simulink model "ECE595_Part1_Project_Lidar_based_Motor_Control_Slave"  (R2017a)
settings: Solver=FixedStepDiscrete  StartTime=0.0  StopTime=10  FixedStep=dt  RelTol=1e-3
InitFcn:
  | mbd_s32k14_consistency_checks(bdroot(gcs));
model workspace (MAT data in the model file):
  MCOS : class17 (value not decoded)
undefined symbols (not defined in the file): A10, AD12, AD6, AD7, Aligned, B10, B8, B9, C10, C7, C8, C9, D1, D2, D8, Edge, External, G2, G3, G5, G6, H8, K10, K5, PTA1, PTA2, PTA3, PTB10, PTB11, PTB12, PTB8, PTB9, PTC10, PTC11, PTC14, PTC6, PTC7, PTD10, PTD11, PTD15, PTD16, PTD4, PTE4, PTE5, SpeedControllerIntegGain, SpeedControllerPropGain, TRGMUX_PDB_TRIG
libraries: mbd_s32k14_ec_toolbox x35, simulink x9
(part 2 of 2)

== system ECE595_Part1_Project_Lidar_based_Motor_Control_Slave/RX_Complete_Event/Switch Case Action Subsystem Data 4 ==
  Action Port : ActionPort  ActionType=case
  Constant : Constant  Value=800  OutDataTypeStr=int16
  Data Store Write : DataStoreWrite  DataStoreName=MotorSpeedReqFreemaster
  FCAN_Receive_ID_0x3FF : mbd_s32k14_ec_toolbox/S32K14x/Communication Blocks/Flex CAN Blocks/FCAN_Receive  can_instance=0  can_mode=Non-blocking  can_timeout_ms=0  can_mb_idx=14  can_extended_id=off  can_is_remote=off  can_id=3FF  can_msg_mask=FFFFFFFF  show_adv_opts=on  can_use_rxfifo=off  can_fd_enable=on
  wires:
  Constant/1 -> Data Store Write/1

== system ECE595_Part1_Project_Lidar_based_Motor_Control_Slave/RX_Complete_Event/Switch Case Action Subsystem Data 5 ==
  Action Port : ActionPort  ActionType=case
  Constant : Constant  Value=800  OutDataTypeStr=int16
  Data Store Write : DataStoreWrite  DataStoreName=MotorSpeedReqFreemaster
  FCAN_Receive_ID_0x3FF : mbd_s32k14_ec_toolbox/S32K14x/Communication Blocks/Flex CAN Blocks/FCAN_Receive  can_instance=0  can_mode=Non-blocking  can_timeout_ms=0  can_mb_idx=14  can_extended_id=off  can_is_remote=off  can_id=3FF  can_msg_mask=FFFFFFFF  show_adv_opts=on  can_use_rxfifo=off  can_fd_enable=on
  wires:
  Constant/1 -> Data Store Write/1

== system ECE595_Part1_Project_Lidar_based_Motor_Control_Slave/RX_Complete_Event/Switch Case Action Subsystem Data 6 ==
  Action Port : ActionPort  ActionType=case
  Constant : Constant  Value=800  OutDataTypeStr=int16
  Data Store Write : DataStoreWrite  DataStoreName=MotorSpeedReqFreemaster
  FCAN_Receive_ID_0x3FF : mbd_s32k14_ec_toolbox/S32K14x/Communication Blocks/Flex CAN Blocks/FCAN_Receive  can_instance=0  can_mode=Non-blocking  can_timeout_ms=0  can_mb_idx=14  can_extended_id=off  can_is_remote=off  can_id=3FF  can_msg_mask=FFFFFFFF  show_adv_opts=on  can_use_rxfifo=off  can_fd_enable=on
  wires:
  Constant/1 -> Data Store Write/1

== system ECE595_Part1_Project_Lidar_based_Motor_Control_Slave/RX_Complete_Event/Switch Case Action Subsystem Data 7 ==
  Action Port : ActionPort  ActionType=case
  Constant : Constant  Value=800  OutDataTypeStr=int16
  Data Store Write : DataStoreWrite  DataStoreName=MotorSpeedReqFreemaster
  FCAN_Receive_ID_0x3FF : mbd_s32k14_ec_toolbox/S32K14x/Communication Blocks/Flex CAN Blocks/FCAN_Receive  can_instance=0  can_mode=Non-blocking  can_timeout_ms=0  can_mb_idx=14  can_extended_id=off  can_is_remote=off  can_id=3FF  can_msg_mask=FFFFFFFF  show_adv_opts=on  can_use_rxfifo=off  can_fd_enable=on
  wires:
  Constant/1 -> Data Store Write/1

== system ECE595_Part1_Project_Lidar_based_Motor_Control_Slave/CalculateRPM/Actual Motor Speed Calculation/Calc_RPM1 ==
  note: Multiply by time constant to get Second
      | Mulitply by 60 to get Minute
      | Divide By State Changes to get Electrical RPM
      | Divide By Pole-Pair to get Mechanical RPM
  HallChangeSum : Inport
  Dir : Inport  Port=2
  GetDirection : Product  Inputs=**  OutDataTypeStr=int16  RndMeth=Zero
  State Changes to RPM Constant : Constant  Value=((1/(dt*250))*60)/(6*4)  OutDataTypeStr=uint16
  TransPerMin : Product  Inputs=**  OutDataTypeStr=uint16  RndMeth=Zero
  RPM : Outport
  wires:
  Dir/1 -> GetDirection/2
  GetDirection/1 -> RPM/1  "MotorSpeedRPM"
  State Changes to RPM Constant/1 -> TransPerMin/2
  HallChangeSum/1 -> TransPerMin/1
  TransPerMin/1 -> GetDirection/1

== system ECE595_Part1_Project_Lidar_based_Motor_Control_Slave/Event_Control/ControlEventLogic/HallChangeCount ==
  function : TriggerPort  TriggerType=function-call  VariantControl=Variant
  Constant5 : Constant  OutDataTypeStr=uint16
  Data Store Read : DataStoreRead  DataStoreName=HallStateChangeDelta
  Data Store Write : DataStoreWrite  DataStoreName=HallStateChangeDelta
  Function-Call Generator : simulink/Ports & Subsystems/Function-Call Generator  sample_time=-1  numberOfIterations=1
  Increment : Sum
  Call : Outport
  wires:
  Increment/1 -> Data Store Write/1
  Constant5/1 -> Increment/1
  Data Store Read/1 -> Increment/2
  Function-Call Generator/1 -> Call/1

== system ECE595_Part1_Project_Lidar_based_Motor_Control_Slave/Event_Control/ControlEventLogic/ToggleLED_HallA ==
  function : TriggerPort  TriggerType=function-call  VariantControl=Variant
  Data Store Read1 : DataStoreRead  DataStoreName=HallInputA
  Data Store Write1 : DataStoreWrite  DataStoreName=HallInputA
  Function-Call Generator : simulink/Ports & Subsystems/Function-Call Generator  sample_time=-1  numberOfIterations=1
  Logical Operator : Logic  Operator=NOT  AllPortsSameDT=off  OutDataTypeStr=boolean
  Call : Outport
  wires:
  Function-Call Generator/1 -> Call/1
  Data Store Read1/1 -> Logical Operator/1
  Logical Operator/1 -> Data Store Write1/1

== system ECE595_Part1_Project_Lidar_based_Motor_Control_Slave/Event_Control/ControlEventLogic/ToggleLED_HallB ==
  function : TriggerPort  TriggerType=function-call  VariantControl=Variant
  Data Store Read1 : DataStoreRead  DataStoreName=HallInputB
  Data Store Write1 : DataStoreWrite  DataStoreName=HallInputB
  Function-Call Generator : simulink/Ports & Subsystems/Function-Call Generator  sample_time=-1  numberOfIterations=1
  Logical Operator : Logic  Operator=NOT  AllPortsSameDT=off  OutDataTypeStr=boolean
  Call : Outport
  wires:
  Function-Call Generator/1 -> Call/1
  Data Store Read1/1 -> Logical Operator/1
  Logical Operator/1 -> Data Store Write1/1

== system ECE595_Part1_Project_Lidar_based_Motor_Control_Slave/Event_Control/ControlEventLogic/ToggleLED_HallC ==
  function : TriggerPort  TriggerType=function-call  VariantControl=Variant
  Data Store Read1 : DataStoreRead  DataStoreName=HallInputC
  Data Store Write1 : DataStoreWrite  DataStoreName=HallInputC
  Function-Call Generator : simulink/Ports & Subsystems/Function-Call Generator  sample_time=-1  numberOfIterations=1
  Logical Operator : Logic  Operator=NOT  AllPortsSameDT=off  OutDataTypeStr=boolean
  Call : Outport
  wires:
  Function-Call Generator/1 -> Call/1
  Data Store Read1/1 -> Logical Operator/1
  Logical Operator/1 -> Data Store Write1/1

== stateflow chart ECE595_Part1_Project_Lidar_based_Motor_Control_Slave/CalculateRPM/Actual Motor Speed Calculation/GatherNumberOfHallStateChanges ==
  (default) -> (junction 5)
  (junction 5) -> (junction 6) : {
      | 	HallChangesSum = HallChangesSum - StoreHallChanges[i];
      | 	StoreHallChanges[i] = HallChanges;
      | 	HallChangesSum = HallChangesSum + StoreHallChanges[i];
      | 	i++;
      | }
  (junction 6) -> (junction 22) [order 2] : {
      | 	HallChangeClear = 0;
      | }
  (junction 6) -> (junction 6) [order 1] : [i >= 250]
      | {i=0;}
  data: StoreHallChanges local uint8 size=[250]; HallChanges input; HallChangesSum output uint16; i local uint8; HallChangeClear output

== stateflow chart ECE595_Part1_Project_Lidar_based_Motor_Control_Slave/Control_Logic/FET pre-driver Initialization Sequence ==
  settings: sampleTime=0.500
  state A
  state B
  state C
  state C1
  state C2
  state D
  state E
  state F
    F -> F [order 1] : {index++;}
  state END
  (default) -> A : {enable=0;}
  A -> B : /*MASK0*/
      | {MPC_Data = 0x20;}
  B -> C : /*MASK1*/
      | {MPC_Data = 0x30;}
  C -> C1 : /*CLINT0*/
      | {MPC_Data = 0x6F;}
  C1 -> C2 : /*CLINT1*/
      | {MPC_Data = 0x7F;}
  C2 -> D : /*Mode*/
      | {MPC_Data  = 0x48;}
  D -> E : {MPC_Data = 0x00;
      | enable=1;}
  E -> F : {Charge_Bootstrap_Low_On;
      | index=0;}
  F -> END [order 1] : [index > 0]
      | {Charge_Bootstrap_All_Off;}
  END -> END : {Normal_Op;
      | MPC_Data = MPC_Cmd;}
  data: MPC_Data output uint16; enable output boolean; index local double; MPC_Cmd data_store_memory
  events: Charge_Bootstrap_Low_On output FUNCTION_CALL_EVENT; Charge_Bootstrap_All_Off output FUNCTION_CALL_EVENT; Normal_Op output FUNCTION_CALL_EVENT

== stateflow chart ECE595_Part1_Project_Lidar_based_Motor_Control_Slave/Event_Control/ControlPollingLogic ==
  state Logic1
    Logic1 -> (junction 25)
    (default) -> (junction 25)
    (junction 25) -> (junction 26) [order 1] : [(MotorSpeedRPM <= 100) && (MotorSpeedRPM >= -100)]
        | {Trigger;}
    (junction 25) -> (junction 28) [order 2]
    (junction 26) -> (junction 27)
    (junction 28) -> (junction 27)
  (default) -> Logic1
  data: MotorSpeedRPM input
  events: Trigger output FUNCTION_CALL_EVENT

== stateflow chart ECE595_Part1_Project_Lidar_based_Motor_Control_Slave/Event_Control/Init ==
  settings: sampleTime=0.500
  state A
  state B
  (default) -> A
  A -> B : {Init;
      | index=0;}
  B -> B
  data: index local double
  events: Init output FUNCTION_CALL_EVENT

== stateflow chart ECE595_Part1_Project_Lidar_based_Motor_Control_Slave/Trapezoidal_Commutation/CommutationTableLookup ==
  (junction 5) -> (junction 15) [order 1] : /*If Direction is Negative */
      | [Direction == -1]
  (default) -> (junction 5)
  (junction 15) -> (junction 14) : {
      |    Phase_A = ccwTable[HallState][0];
      |    Phase_B = ccwTable[HallState][1];
      |    Phase_C = ccwTable[HallState][2];
      | }
  (junction 5) -> (junction 6) [order 2] : {
      |    Phase_A = cwTable[HallState][0];
      |    Phase_B = cwTable[HallState][1];
      |    Phase_C = cwTable[HallState][2];
      | }
  (junction 6) -> (junction 14)
  data: cwTable constant uint8 size=[8 3] =[0 0 0; 2 1 0; 0 2 1; 2 0 1; 1 0 2; 0 1 2; 1 2 0; 0 0 0]; HallState input; Phase_A output uint8; Phase_B output uint8; Phase_C output uint8; ccwTable constant uint8 size=[8 3] =[0 0 0; 1 2 0; 0 1 2; 1 0 2; 2 0 1; 0 2 1; 2 1 0; 0 0 0]; Direction input

== stateflow chart ECE595_Part1_Project_Lidar_based_Motor_Control_Slave/Trapezoidal_Commutation/PhaseSwitchLogic ==
  settings: sampleTime=0.500
  note: Phase States:
      | 0 = NC
      | 1 = -Vdcb
      | 2 = +Vdcb
  (default) -> (junction 13)
  (junction 13) -> (junction 14) [order 1] : /*check for phase state 0 */
      | [Phase_A == 0]
      | /*set output for state 0 */
      | {Phase_A_HS = 0; Phase_A_LS =0;}
  (junction 13) -> (junction 17) [order 2]
  (junction 14) -> (junction 16)
  (junction 17) -> (junction 16) [order 1] : /*check for phase state 1 */
      | [Phase_A == 1]
      | /*set output for state 1 */
      | {Phase_A_HS = 0; Phase_A_LS = PWM_Duty_Cycle;}
  (junction 17) -> (junction 20) [order 2]
  (junction 16) -> (junction 19)
  (junction 20) -> (junction 19) [order 1] : /*check for phase state 2 */
      | [Phase_A == 2]
      | /*set output for state 2 */
      | {Phase_A_HS = 1000; Phase_A_LS = 0;}
  (junction 20) -> (junction 62) [order 2]
  (junction 19) -> (junction 23)
  (junction 62) -> (junction 23)
  (junction 23) -> (junction 22) [order 1] : /*check for phase state 0 */
      | [Phase_B == 0]
      | /*set output for state 0 */
      | {Phase_B_HS = 0; Phase_B_LS = 0;}
  (junction 23) -> (junction 26) [order 2]
  (junction 22) -> (junction 25)
  (junction 26) -> (junction 25) [order 1] : /*check for phase state 1 */
      | [Phase_B == 1]
      | /*set output for state 1 */
      | {Phase_B_HS = 0; Phase_B_LS = PWM_Duty_Cycle;}
  (junction 26) -> (junction 29) [order 2]
  (junction 25) -> (junction 28)
  (junction 29) -> (junction 28) [order 1] : /*check for phase state 2 */
      | [Phase_B == 2]
      | /*set output for state 2 */
      | {Phase_B_HS = 1000; Phase_B_LS = 0;}
  (junction 29) -> (junction 65) [order 2]
  (junction 28) -> (junction 49)
  (junction 65) -> (junction 49)
  (junction 49) -> (junction 48) [order 1] : /*check for phase state 0 */
      | [Phase_C == 0]
      | /*set output for state 0 */
      | {Phase_C_HS = 0; Phase_C_LS = 0;}
  (junction 49) -> (junction 51) [order 2]
  (junction 48) -> (junction 50)
  (junction 51) -> (junction 50) [order 1] : /*check for phase state 1 */
      | [Phase_C == 1]
      | /*set output for state 1 */
      | {Phase_C_HS = 0; Phase_C_LS = PWM_Duty_Cycle;}
  (junction 51) -> (junction 53) [order 2]
  (junction 50) -> (junction 52)
  (junction 53) -> (junction 52) [order 1] : /*check for phase state 2 */
      | [Phase_C == 2]
      | /*set output for state 2 */
      | {Phase_C_HS = 1000; Phase_C_LS = 0;}
  (junction 53) -> (junction 70) [order 2]
  (junction 52) -> (junction 69)
  (junction 70) -> (junction 69)
  data: Phase_A input; Phase_B input; Phase_C input; Phase_A_HS output uint32; Phase_A_LS output uint32; Phase_B_HS output uint32; Phase_B_LS output uint32; Phase_C_HS output uint32; Phase_C_LS output uint32; PWM_Duty_Cycle input
